simulink model "Sim_tracking_1_3_4"  (R2024b)
settings: Solver=VariableStepAuto  StartTime=0.0  StopTime=T_SIM  MaxStep=0.001  RelTol=1e-3
values from neighbouring files (symbols this model uses):
  d_actual = 0.165    [data_for_identification.mat]    (also in id_template.m; init_localization.m = 0.164; init_localization_template.m = 0.164; script_init_localization.m = 0.164)
  Q_INIT = [0 0 0.463647609001]    [data_for_identification.mat]    (also in id_LEO.m = q(:,1); id_template.m = [0;0;atan(0.5)]; init_localization.m = [0;0;0]; script_init_localization.m = q(:,1))
  r_actual = 0.03    [data_for_identification.mat]    (also in id_template.m; init_localization.m = 0.031; init_localization_template.m = 0.031; script_init_localization.m = 0.031)
  T_s = Ts_values(i)    [EX_opt_1.m]    (also in EX_opt_2.m; data_for_identification.mat = 0.04; id_LEO.m = 0.04; id_template.m = 0.04)
settings Model: Creator=alberto  LastModifiedBy=loren
settings RTWCC: GPUComputeCapability=3.5
settings ConfigComp: CovBoundaryAbsTol=1.0e-5

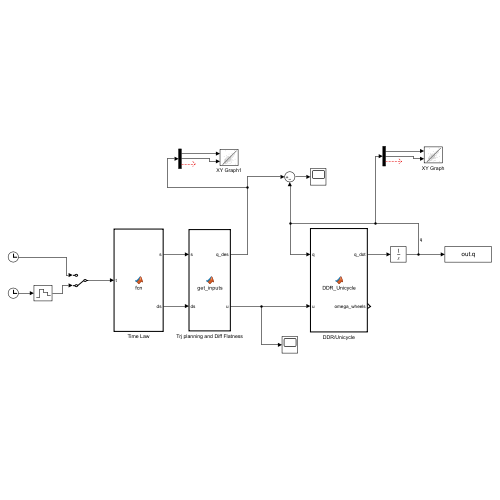
[thumbnail: Simulink's stored preview of the top-level diagram]
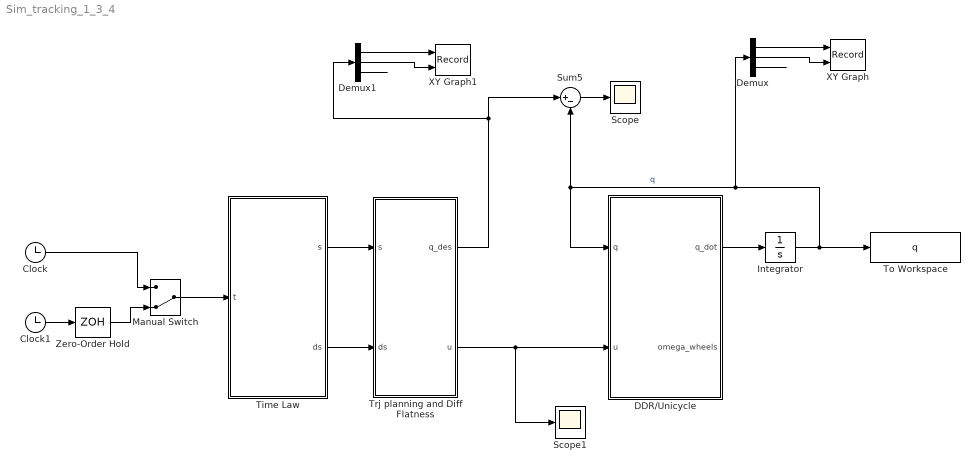
== system Sim_tracking_1_3_4 ==
  Clock : Clock
  Clock1 : Clock
  DDR/Unicycle : MATLAB Function  TreatAsAtomicUnit=on
  Demux : Demux  Outputs=3
  Demux1 : Demux  Outputs=3
  Integrator : Integrator  InitialCondition=Q_INIT
  Manual Switch : ManualSwitch  CurrentSetting=0
  Scope : Scope
  Scope1 : Scope
  Sum5 : Sum  Inputs=|+-
  Time Law : MATLAB Function  TreatAsAtomicUnit=on
  To Workspace : ToWorkspace  VariableName=q  SaveFormat=Structure With Time  SampleTime=-1
  Trj planning and Diff Flatness : MATLAB Function  TreatAsAtomicUnit=on
  XY Graph : Record  FileSettingsInternal="{\"entries\":[{\"content\":{\"excelSettings\":{\"content\":{},\"type\":\"Streamout.ExcelSettings\"},\"parquetSettings\":{\"content\":{},\"type\":\"Streamout.ParquetSettings\"}},\"type\":\"Streamout.FileSettingStorage\",\"uuid\":\"\"}],\"packageUris\":[\"http:\\/\\/schema.mathworks.com\\/mf0\\/streamout_blocks\\/R2020a\"],\"version\":\"1.0\"}"  Layout=[1 1]  SignalsInternal="{\"entries\":[{\"content\":{\"signals\":[{\"content\":{\"blockPath\":[],\"dimensions\":[1,1],\"domain\":\"\",\"lineColor\":\"#a2142f\",\"plots\":[ 1 ],\"port\":1,\"signalID\":1,\"signalName\":\"Demux:1\"},\"type\":\"RecordBlkView.Signal\",\"uuid\":\"\"},{\"content\":{\"blockPath\":[],\"dimensions\":[1,1],\"domain\":\"\",\"lineColor\":\"#139fff\",\"plots\":[ 1 ],\"port\":2,\"signalID\":2,\"signalName\":\"Demux:2\"},\"type\":\"RecordBlkView.Signal\",\"uuid\":\"\"}]},\"type\":\"RecordBlkView.InputSignals\",\"uuid\":\"\"}],\"packageUris\":[\"http:\\/\\/schema.mathworks.com\\/mf0\\/streamout_blocks\\/R2020a\"],\"version\":\"1.0\"}"  VisualizationBindings="{\"xyplotplugin\":{\"info\":[{\"series\":[{\"bindingParametersList\":[{\"parameter\":\"X-Axis\",\"signalID\":1,\"signalName\":\"Demux:1\"},{\"parameter\":\"Y-Axis\",\"signalID\":2,\"signalName\":\"Demux:2\"}],\"seriesID\":0}],\"subplotID\":1}]}}"  CompatibilityTag=XY
  XY Graph1 : Record  FileSettingsInternal="{\"entries\":[{\"content\":{\"excelSettings\":{\"content\":{},\"type\":\"Streamout.ExcelSettings\"},\"parquetSettings\":{\"content\":{},\"type\":\"Streamout.ParquetSettings\"}},\"type\":\"Streamout.FileSettingStorage\",\"uuid\":\"\"}],\"packageUris\":[\"http:\\/\\/schema.mathworks.com\\/mf0\\/streamout_blocks\\/R2020a\"],\"version\":\"1.0\"}"  Layout=[1 1]  SignalsInternal="{\"entries\":[{\"content\":{\"signals\":[{\"content\":{\"blockPath\":[],\"dimensions\":[1,1],\"domain\":\"\",\"lineColor\":\"#a2142f\",\"plots\":[ 1 ],\"port\":1,\"signalID\":1,\"signalName\":\"Demux1:1\"},\"type\":\"RecordBlkView.Signal\",\"uuid\":\"\"},{\"content\":{\"blockPath\":[],\"dimensions\":[1,1],\"domain\":\"\",\"lineColor\":\"#139fff\",\"plots\":[ 1 ],\"port\":2,\"signalID\":2,\"signalName\":\"Demux1:2\"},\"type\":\"RecordBlkView.Signal\",\"uuid\":\"\"}]},\"type\":\"RecordBlkView.InputSignals\",\"uuid\":\"\"}],\"packageUris\":[\"http:\\/\\/schema.mathworks.com\\/mf0\\/streamout_blocks\\/R2020a\"],\"version\":\"1.0\"}"  VisualizationBindings="{\"xyplotplugin\":{\"info\":[{\"series\":[{\"bindingParametersList\":[{\"parameter\":\"X-Axis\",\"signalID\":1,\"signalName\":\"Demux1:1\"},{\"parameter\":\"Y-Axis\",\"signalID\":2,\"signalName\":\"Demux1:2\"}],\"seriesID\":0}],\"subplotID\":1}]}}"  CompatibilityTag=XY
  Zero-Order Hold : ZeroOrderHold  SampleTime=T_s
  wires:
  Manual Switch/1 -> Time Law/1(t)
  Clock1/1 -> Zero-Order Hold/1
  Demux/2 -> XY Graph/2
  Time Law/1(s) -> Trj planning and Diff Flatness/1(s)
  Trj planning and Diff Flatness/2(u) -> Scope1/1, DDR/Unicycle/2(u)
  Time Law/2(ds) -> Trj planning and Diff Flatness/2(ds)
  DDR/Unicycle/1(q_dot) -> Integrator/1
  Trj planning and Diff Flatness/1(q_des) -> Sum5/1, Demux1/1
  Demux1/2 -> XY Graph1/2
  Demux1/1 -> XY Graph1/1
  Demux/3 -> ?
  Zero-Order Hold/1 -> Manual Switch/2
  Demux1/3 -> ?
  Clock/1 -> Manual Switch/1
  Sum5/1 -> Scope/1
  Integrator/1 -> To Workspace/1, Demux/1, Sum5/2, DDR/Unicycle/1(q)  "q"
  Demux/1 -> XY Graph/1

== matlab function Sim_tracking_1_3_4/Time Law ==
  data: t input; s output; ds output
function [s, ds] = fcn(t)
    
    Ta = 0.5;
    Tc = 9; 
        
    vc = 1/(Ta+Tc);
    a = vc/Ta;
   
    if t < Ta
        s_dot = a*t;
        s = 0.5*a*t^2;
    
    elseif t < (Ta+Tc)
        s_dot = vc;
        s = 0.5*a*Ta^2 + vc*(t - Ta);
    
    elseif t < (2*Ta+Tc)
        s_dot = vc - a*(t - Ta - Tc);
        s = 0.5*a*Ta^2 + vc*Tc + vc*(t - Ta - Tc) ...
            - 0.5*a*(t - Ta - Tc)^2;
    else
        s_dot = 0;
        s = 1;
    end

    ds = s_dot;
    
end

== matlab function Sim_tracking_1_3_4/DDR//Unicycle ==
  data: q input; u input; q_dot output; omega_wheels output; d_actual parameter; r_actual parameter
function [q_dot, omega_wheels] = DDR_Unicycle(q, u, d_actual, r_actual)

    % extract variables
    v = u(1);
    omega = u(2);

    q_dot= zeros(3,1);
    
    q_dot(1) = v*cos(q(3));
    q_dot(2) = v*sin(q(3));
    q_dot(3) = omega;

    
    wL = v/r_actual - d_actual/(2*r_actual) * omega;
    wR = v/r_actual + d_actual/(2*r_actual) * omega;

    omega_wheels = [wL, wR];

end

== matlab function Sim_tracking_1_3_4/Trj planning and Diff Flatness ==
  data: q_des output; s input; u output; ds input
function [q_des, u] = get_inputs(s, ds)

    R = 0.4;
    w = 2*pi;

    % function [x_s, y_s, x_s_dot, y_s_dot, x_s_ddot, y_s_ddot] = gen_eight_shape_trajectory(R, w, s)
   
    x_s = R*sin(2*w*s);
    y_s = R*sin(w*s);
    
    % computes derivatives analytically

    x_s_dot = 2*R*w*cos(2*w*s);
    y_s_dot = R*w*cos(w*s);
    
    x_s_ddot = -4*R*w^2*sin(2*w*s);
    y_s_ddot = -R*w^2*sin(w*s);


    % function [q, u] = flat_to_kinematic_cartesian(x, y, x_dot, y_dot, x_ddot, y_ddot)

    theta = atan2(y_s_dot, x_s_dot);
    
    q_des = [x_s; y_s; theta];
   
    v_tilde = sqrt(x_s_dot^2 + y_s_dot^2);
    omega_tilde = (x_s_dot * y_s_ddot - y_s_dot * x_s_ddot) / (x_s_dot^2 + y_s_dot^2);
    
    % Convert into real Inputs
    v = v_tilde * ds;
    omega = omega_tilde * ds;
    
    u = [v; omega];
end
